simulink library "partitionedLifitngBdy_cls"  (R2018b)
settings: Solver=VariableStepAuto  StartTime=0.0  StopTime=10.0  RelTol=1e-3
undefined symbols (not defined in the file or in its folder): env_t, tp
libraries: BdyFrameGravForce_ul x1, bdyFrameBuoyFnM_ul x1, calcAttchPtStates_ul x1, partitionedLifitngBdy_cl x1, simpleDragTurbine_ul x1, sixDoFDynamics_ul x1, sumAttchPtsFnM_ul x1
settings Model: Creator=Ayaz  LastModifiedBy=asiddiq2

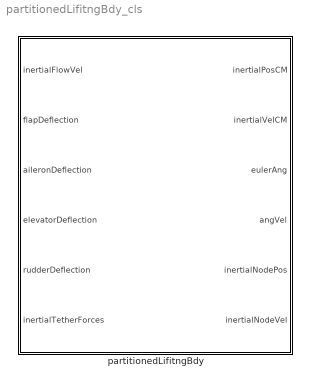
== system partitionedLifitngBdy_cls ==
  partitionedLifitngBdy : Subsystem  mask{M=tp.vehicle.mass.value, M_added=tp.vehicle.added_mass.value, J=tp.vehicle.MI.value, vol=tp.vehicle.volume.value, Rcb_cm=tp.vehicle.Rcb_cm.value, tb=tp.turbines, atp=tp.vehicleTetherAttchPts, g=tp.vehicle.mass.value, rho_fluid=env_t.flowDensity.value, aero_struct=tp.aeroCoeffData, initPos=tp.vehicle.ini_Rcm_o.value, initVel=tp.vehicle.ini_O_Vcm_o.value, initEulAngs=tp.vehicle.ini_euler.value, initAngVel=tp.vehicle.ini_OwB.value}
      mask prompts: M "Mass"; M_added "Added Mass Matrix"; J "Inertia matrix"; vol "Body volume"; Rcb_cm "Center of buoyamcy vector"; tb "Turbines structure"; atp "Attachment point structure"; g "Gravitational acceleration"; rho_fluid "Fluid density"; aero_struct "Structure containing AVL data"; initPos "Initial position"; initVel "Initial velocity"; initEulAngs "Initial Euler Angles"; initAngVel "Initial Angular Velocity Vec"
      mask TypeOptions M: BdyFrameGravForce/M | sixDoFDynamics1/M
      mask TypeOptions M_added: sixDoFDynamics1/M_added
      mask TypeOptions J: sixDoFDynamics1/J
      mask TypeOptions vol: bdyFrameBuoyForceAndMoment/vol
      mask TypeOptions Rcb_cm: bdyFrameBuoyForceAndMoment/Rcb_cm
      mask TypeOptions tb: simpleDragTurbine/tb
      mask TypeOptions atp: sumAttchPtsFnM/atp | calcAttchPtStates/atp
      mask TypeOptions g: BdyFrameGravForce/g | bdyFrameBuoyForceAndMoment/g
      mask TypeOptions rho_fluid: bdyFrameBuoyForceAndMoment/rho_fluid | simpleDragTurbine/rho_fluid | partitionedLiftingBdy/rho_fluid
      mask TypeOptions aero_struct: partitionedLiftingBdy/aero_struct
      mask TypeOptions initPos: sixDoFDynamics1/initPos
      mask TypeOptions initVel: sixDoFDynamics1/initVel
      mask TypeOptions initEulAngs: sixDoFDynamics1/initEulAngs
      mask TypeOptions initAngVel: sixDoFDynamics1/initAngVel
      mask DialogControl Container20 Prompt: Parameters
      mask DialogControl ParameterGroupVar Prompt: Physical Parameters
      mask DialogControl Container12 Prompt: Turbine
      mask DialogControl Container13 Prompt: Tether attachment points
      mask DialogControl Container24 Prompt: Environment
      mask DialogControl Container11 Prompt: Fluid Dynamic Surface
      mask DialogControl Container25 Prompt: Initial conditions

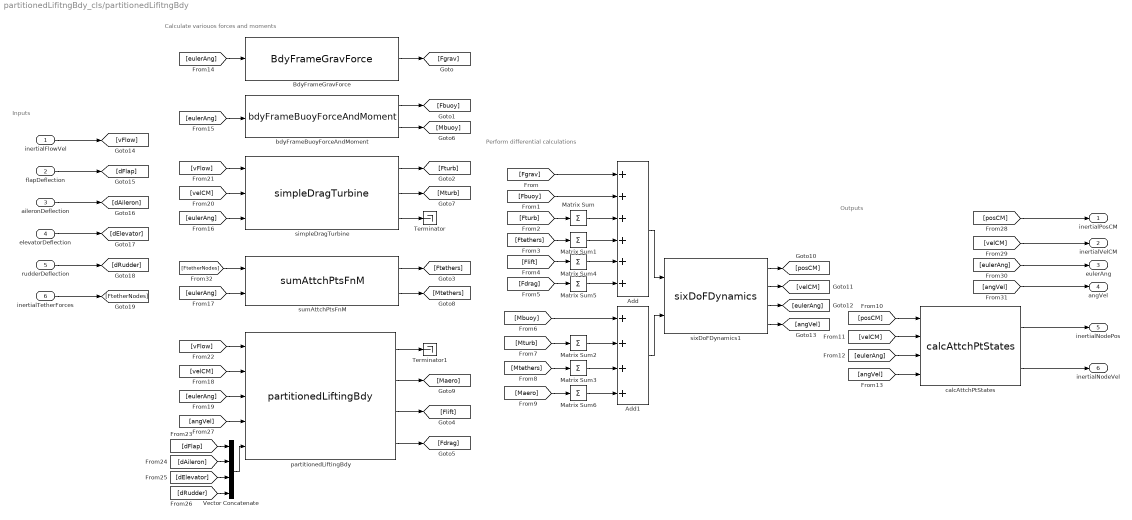
== system partitionedLifitngBdy_cls/partitionedLifitngBdy ==
  note: Outputs
  note: Inputs
  note: Calculate variouos forces and moments
  note: Perform differential calculations
  inertialFlowVel : Inport
  flapDeflection : Inport  Port=2
  aileronDeflection : Inport  Port=3
  elevatorDeflection : Inport  Port=4
  rudderDeflection : Inport  Port=5
  inertialTetherForces : Inport  Port=6
  Add : Sum  Inputs=++++++
  Add1 : Sum  Inputs=++++
  BdyFrameGravForce : BdyFrameGravForce_ul/BdyFrameGravForce  M=M  g=g
  Matrix Sum{,1..6} (7 alike) : Sum  Inputs=+  CollapseMode=Specified dimension  CollapseDim=2
  Terminator : Terminator
  Terminator1 : Terminator
  Vector Concatenate : Concatenate  NumInputs=4
  bdyFrameBuoyForceAndMoment : bdyFrameBuoyFnM_ul/bdyFrameBuoyForceAndMoment  vol=vol  rho_fluid=rho_fluid  g=g  Rcb_cm=Rcb_cm
  calcAttchPtStates : calcAttchPtStates_ul/calcAttchPtStates  atp=atp
  partitionedLiftingBdy : partitionedLifitngBdy_cl/partitionedLiftingBdy  rho_fluid=rho_fluid  aero_struct=aero_struct
  simpleDragTurbine : simpleDragTurbine_ul/simpleDragTurbine  rho_fluid=rho_fluid  tb=tb
  sixDoFDynamics1 : sixDoFDynamics_ul/sixDoFDynamics  M=M  M_added=M_added  J=J  initPos=initPos  initVel=initVel  initEulAngs=initEulAngs  initAngVel=initAngVel
  sumAttchPtsFnM : sumAttchPtsFnM_ul/sumAttchPtsFnM  atp=atp
  inertialPosCM : Outport
  inertialVelCM : Outport  Port=2
  eulerAng : Outport  Port=3
  angVel : Outport  Port=4
  inertialNodePos : Outport  Port=5
  inertialNodeVel : Outport  Port=6
  wires:
  [Mtethers] -> Matrix Sum3/1
  [velCM] -> partitionedLiftingBdy/2
  [angVel] -> calcAttchPtStates/4
  [eulerAng] -> calcAttchPtStates/3
  sixDoFDynamics1/4 -> [angVel]
  sixDoFDynamics1/3 -> [eulerAng]
  [posCM] -> calcAttchPtStates/1
  sixDoFDynamics1/2 -> [velCM]
  [Mturb] -> Matrix Sum2/1
  [eulerAng] -> sumAttchPtsFnM/2
  [eulerAng] -> bdyFrameBuoyForceAndMoment/1
  [eulerAng] -> BdyFrameGravForce/1
  [Mbuoy] -> Add1/1
  simpleDragTurbine/3 -> Terminator/1
  [Ftethers] -> Matrix Sum1/1
  partitionedLiftingBdy/4 -> [Fdrag]
  Add1/1 -> sixDoFDynamics1/2
  partitionedLiftingBdy/2 -> [Maero]
  [Fbuoy] -> Add/2
  partitionedLiftingBdy/3 -> [Flift]
  sumAttchPtsFnM/1 -> [Ftethers]
  [velCM] -> calcAttchPtStates/2
  [Maero] -> Matrix Sum6/1
  [Fturb] -> Matrix Sum/1
  simpleDragTurbine/2 -> [Mturb]
  simpleDragTurbine/1 -> [Fturb]
  [Flift] -> Matrix Sum4/1
  Add/1 -> sixDoFDynamics1/1
  bdyFrameBuoyForceAndMoment/2 -> [Mbuoy]
  [eulerAng] -> partitionedLiftingBdy/3
  BdyFrameGravForce/1 -> [Fgrav]
  [Fdrag] -> Matrix Sum5/1
  [Fgrav] -> Add/1
  sumAttchPtsFnM/2 -> [Mtethers]
  bdyFrameBuoyForceAndMoment/1 -> [Fbuoy]
  [eulerAng] -> simpleDragTurbine/3
  [velCM] -> simpleDragTurbine/2
  sixDoFDynamics1/1 -> [posCM]
  inertialFlowVel/1 -> [vFlow]
  [vFlow] -> simpleDragTurbine/1
  [vFlow] -> partitionedLiftingBdy/1
  rudderDeflection/1 -> [dRudder]
  elevatorDeflection/1 -> [dElevator]
  aileronDeflection/1 -> [dAileron]
  flapDeflection/1 -> [dFlap]
  [dElevator] -> Vector Concatenate/3
  [dRudder] -> Vector Concatenate/4
  inertialTetherForces/1 -> [FtetherNodes]
  [FtetherNodes] -> sumAttchPtsFnM/1
  [posCM] -> inertialPosCM/1
  [velCM] -> inertialVelCM/1
  [eulerAng] -> eulerAng/1
  [angVel] -> angVel/1
  calcAttchPtStates/2 -> inertialNodeVel/1
  calcAttchPtStates/1 -> inertialNodePos/1
  Matrix Sum/1 -> Add/3
  Matrix Sum1/1 -> Add/4
  Matrix Sum2/1 -> Add1/2
  Matrix Sum3/1 -> Add1/3
  [angVel] -> partitionedLiftingBdy/4
  [dFlap] -> Vector Concatenate/1
  [dAileron] -> Vector Concatenate/2
  Vector Concatenate/1 -> partitionedLiftingBdy/5
  Matrix Sum4/1 -> Add/5
  Matrix Sum5/1 -> Add/6
  Matrix Sum6/1 -> Add1/4
  partitionedLiftingBdy/1 -> Terminator1/1
